simulink library "ERR_lib"  (Simulink 7.5)
settings: Solver=ode45  StartTime=0.0  StopTime=10.0  RelTol=1e-3
values from neighbouring files (symbols this model uses):
  pERR_bool_ErrDsblSwt_C = Simulink.Parameter    [ERR_par.m]
  pERR_bool_ErrIntial_C = Simulink.Parameter    [ERR_par.m]
  pERR_st_ACPTCErr_C = Simulink.Parameter    [ERR_par.m]
  pERR_st_HCUErrLampCalSt_C = Simulink.Parameter    [ERR_par.m]
  pERR_st_HCUErrLampEnbl_C = Simulink.Parameter    [ERR_par.m]
  pERR_st_HCUIntialSt_C = Simulink.Parameter    [ERR_par.m]
  pERR_st_HCUStNoErr_C = Simulink.Parameter    [ERR_par.m]
undefined symbols (not defined in the file or in its folder): p_bool_False_M, p_single_Zero_M
libraries: BaseOperationLib_Browser x64, PES_CZ_FAW x56, simulink x2
settings Model: Creator=wuaibin  LastModifiedBy=wuaibin

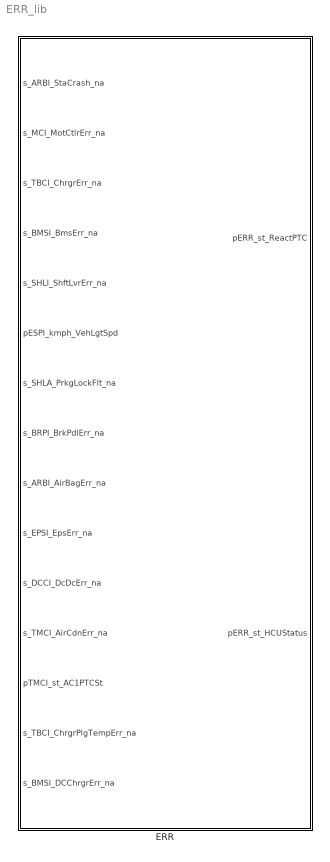
== system ERR_lib ==
  ERR : Subsystem  TreatAsAtomicUnit=on

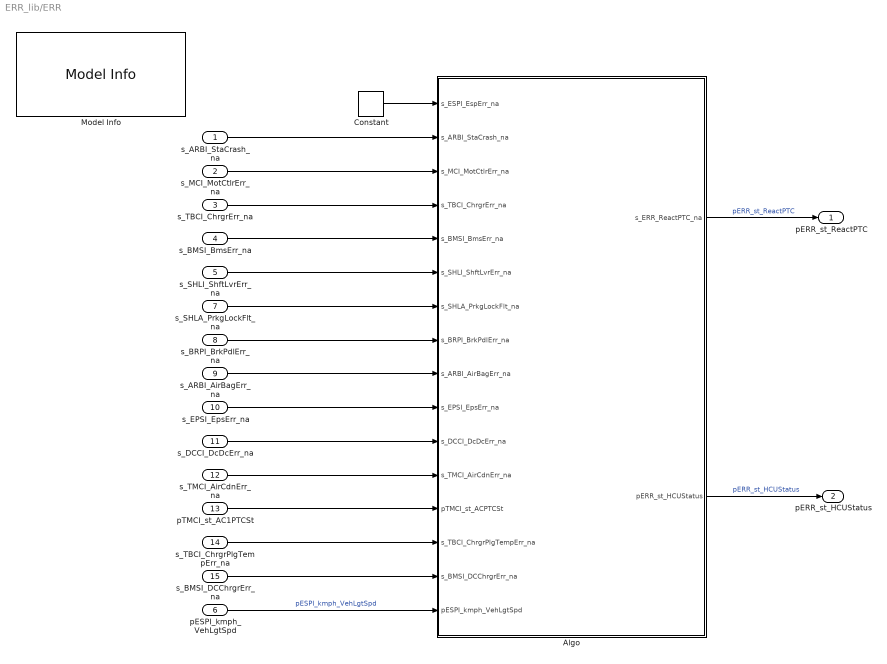
== system ERR_lib/ERR ==
  s_ARBI_StaCrash_na : Inport  PortDimensions=1
  s_MCI_MotCtlrErr_na : Inport  Port=2  PortDimensions=1
  s_TBCI_ChrgrErr_na : Inport  Port=3  PortDimensions=1
  s_BMSI_BmsErr_na : Inport  Port=4  PortDimensions=1
  s_SHLI_ShftLvrErr_na : Inport  Port=5  PortDimensions=1
  pESPI_kmph_VehLgtSpd : Inport  Port=6
  s_SHLA_PrkgLockFlt_na : Inport  Port=7  PortDimensions=1
  s_BRPI_BrkPdlErr_na : Inport  Port=8  PortDimensions=1
  s_ARBI_AirBagErr_na : Inport  Port=9  PortDimensions=1
  s_EPSI_EpsErr_na : Inport  Port=10  PortDimensions=1
  s_DCCI_DcDcErr_na : Inport  Port=11  PortDimensions=1
  s_TMCI_AirCdnErr_na : Inport  Port=12  PortDimensions=1
  pTMCI_st_AC1PTCSt : Inport  Port=13
  s_TBCI_ChrgrPlgTempErr_na : Inport  Port=14
  s_BMSI_DCChrgrErr_na : Inport  Port=15
  Algo : Subsystem
  Constant : BaseOperationLib_Browser/Sources&Sinks/Constant  Value=0  OutMin=[]  OutMax=[]  OutDataTypeMode=uint32  OutDataType=fixdt(1, 16)  ConRadixGroup=Use specified scaling  OutScaling=2^0  OutDataTypeStr=uint32
  Model Info : simulink/Model-Wide Utilities/Model Info  SystemSampleTime=-1  InitialBlockCM=None  BlockCM=None  Frame=on  DisplayStringWithTags=Model Info\nCreated: %<Created>\nCreator: wuaibin  HorizontalTextAlignment=Center  LeftAlignmentValue=0.5  SourceBlockDiagram=HQEV_HCU  TagMaxNumber=20
  pERR_st_ReactPTC : Outport  PortDimensions=1
  pERR_st_HCUStatus : Outport  Port=2
  wires:
  pESPI_kmph_VehLgtSpd/1 -> Algo/16(pESPI_kmph_VehLgtSpd)  "pESPI_kmph_VehLgtSpd"
  Constant/1 -> Algo/1(s_ESPI_EspErr_na)
  s_BMSI_DCChrgrErr_na/1 -> Algo/15(s_BMSI_DCChrgrErr_na)
  s_TBCI_ChrgrPlgTempErr_na/1 -> Algo/14(s_TBCI_ChrgrPlgTempErr_na)
  pTMCI_st_AC1PTCSt/1 -> Algo/13(pTMCI_st_ACPTCSt)
  Algo/2(pERR_st_HCUStatus) -> pERR_st_HCUStatus/1  "pERR_st_HCUStatus"
  s_ARBI_StaCrash_na/1 -> Algo/2(s_ARBI_StaCrash_na)
  s_MCI_MotCtlrErr_na/1 -> Algo/3(s_MCI_MotCtlrErr_na)
  s_TBCI_ChrgrErr_na/1 -> Algo/4(s_TBCI_ChrgrErr_na)
  s_BMSI_BmsErr_na/1 -> Algo/5(s_BMSI_BmsErr_na)
  s_SHLI_ShftLvrErr_na/1 -> Algo/6(s_SHLI_ShftLvrErr_na)
  Algo/1(s_ERR_ReactPTC_na) -> pERR_st_ReactPTC/1  "pERR_st_ReactPTC"
  s_SHLA_PrkgLockFlt_na/1 -> Algo/7(s_SHLA_PrkgLockFlt_na)
  s_BRPI_BrkPdlErr_na/1 -> Algo/8(s_BRPI_BrkPdlErr_na)
  s_ARBI_AirBagErr_na/1 -> Algo/9(s_ARBI_AirBagErr_na)
  s_EPSI_EpsErr_na/1 -> Algo/10(s_EPSI_EpsErr_na)
  s_DCCI_DcDcErr_na/1 -> Algo/11(s_DCCI_DcDcErr_na)
  s_TMCI_AirCdnErr_na/1 -> Algo/12(s_TMCI_AirCdnErr_na)

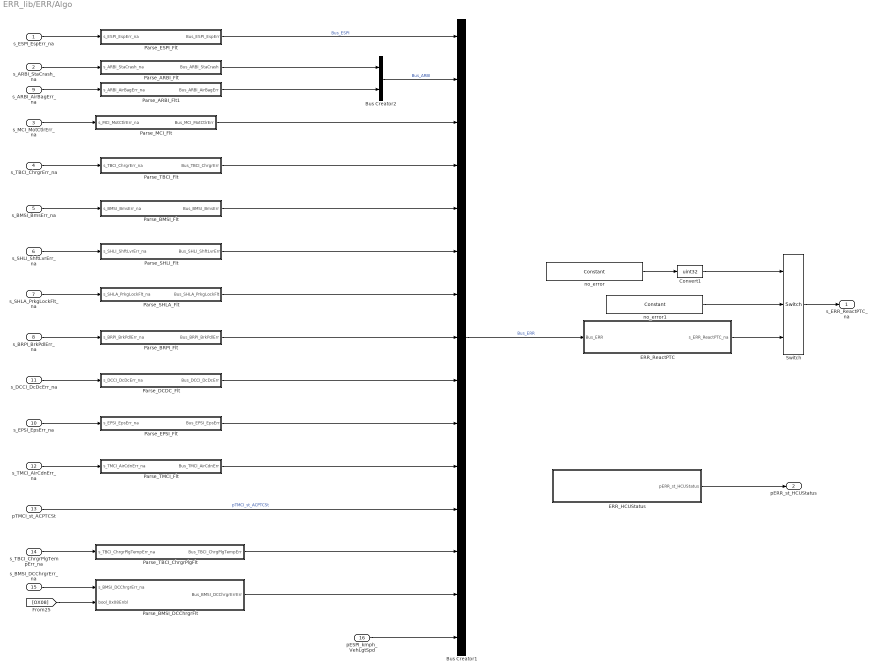
== system ERR_lib/ERR/Algo ==
  s_ESPI_EspErr_na : Inport
  s_ARBI_StaCrash_na : Inport  Port=2
  s_MCI_MotCtlrErr_na : Inport  Port=3
  s_TBCI_ChrgrErr_na : Inport  Port=4
  s_BMSI_BmsErr_na : Inport  Port=5
  s_SHLI_ShftLvrErr_na : Inport  Port=6
  s_SHLA_PrkgLockFlt_na : Inport  Port=7
  s_BRPI_BrkPdlErr_na : Inport  Port=8
  s_ARBI_AirBagErr_na : Inport  Port=9
  s_EPSI_EpsErr_na : Inport  Port=10
  s_DCCI_DcDcErr_na : Inport  Port=11
  s_TMCI_AirCdnErr_na : Inport  Port=12
  pTMCI_st_ACPTCSt : Inport  Port=13
  s_TBCI_ChrgrPlgTempErr_na : Inport  Port=14
  s_BMSI_DCChrgrErr_na : Inport  Port=15
  pESPI_kmph_VehLgtSpd : Inport  Port=16
  Bus Creator1 : BusCreator  Inputs=15
  Bus Creator2 : BusCreator  Inputs=2
  Convert1 : DataTypeConversion  OutDataTypeMode=uint32  OutDataType=fixdt(1, 16)  OutScaling=2^0  OutDataTypeStr=uint32
  ERR_HCUStatus : Subsystem
  ERR_ReactPTC : Subsystem
  Parse_ARBI_Flt : Subsystem
  Parse_ARBI_Flt1 : Subsystem
  Parse_BMSI_DCChrgrFlt : Subsystem
  Parse_BMSI_Flt : Subsystem
  Parse_BRPI_Flt : Subsystem
  Parse_DCDC_Flt : Subsystem
  Parse_EPSI_Flt : Subsystem
  Parse_ESPI_Flt : Subsystem
  Parse_MCI_Flt : Subsystem
  Parse_SHLA_Flt : Subsystem
  Parse_SHLI_Flt : Subsystem
  Parse_TBCI_ChrgrPlgFlt : Subsystem
  Parse_TBCI_Flt : Subsystem
  Parse_TMCI_Flt : Subsystem
  Switch : BaseOperationLib_Browser/Signal Routing Changed/Switch  Criteria=u2 ~= 0  Threshold=0  OutMin=[]  OutMax=[]  OutDataType=fixdt(1,16,0)  OutScaling=[]
  no_error : BaseOperationLib_Browser/Sources&Sinks/Constant  Value=pERR_bool_ErrIntial_C  OutMin=[]  OutMax=[]  OutDataType=fixdt(1, 16)  ConRadixGroup=Use specified scaling  OutScaling=2^0  OutDataTypeStr=Inherit: Inherit from 'Constant value'
  no_error1 : BaseOperationLib_Browser/Sources&Sinks/Constant  Value=pERR_bool_ErrDsblSwt_C  OutMin=[]  OutMax=[]  OutDataType=fixdt(1, 16)  ConRadixGroup=Use specified scaling  OutScaling=2^0  OutDataTypeStr=Inherit: Inherit from 'Constant value'
  s_ERR_ReactPTC_na : Outport
  pERR_st_HCUStatus : Outport  Port=2
  wires:
  pESPI_kmph_VehLgtSpd/1 -> Bus Creator1/15
  Parse_BMSI_DCChrgrFlt/1(Bus_BMSI_DCChrgrErrErr) -> Bus Creator1/14
  Parse_TBCI_ChrgrPlgFlt/1(Bus_TBCI_ChrgPlgTempErr) -> Bus Creator1/13
  [OX08] -> Parse_BMSI_DCChrgrFlt/2(bool_0x08Enbl)
  s_BMSI_DCChrgrErr_na/1 -> Parse_BMSI_DCChrgrFlt/1(s_BMSI_DCChrgrErr_na)
  s_TBCI_ChrgrPlgTempErr_na/1 -> Parse_TBCI_ChrgrPlgFlt/1(s_TBCI_ChrgrPlgTempErr_na)
  pTMCI_st_ACPTCSt/1 -> Bus Creator1/12  "pTMCI_st_ACPTCSt"
  ERR_HCUStatus/1(pERR_st_HCUStatus) -> pERR_st_HCUStatus/1
  Parse_EPSI_Flt/1(Bus_EPSI_EpsErr) -> Bus Creator1/10
  Parse_DCDC_Flt/1(Bus_DCCI_DcDcErr) -> Bus Creator1/9
  Bus Creator2/1 -> Bus Creator1/2  "Bus_ARBI"
  Parse_ARBI_Flt1/1(Bus_ARBI_AirBagErr) -> Bus Creator2/2
  Parse_BRPI_Flt/1(Bus_BRPI_BrkPdlErr) -> Bus Creator1/8
  s_BRPI_BrkPdlErr_na/1 -> Parse_BRPI_Flt/1(s_BRPI_BrkPdlErr_na)
  Parse_SHLA_Flt/1(Bus_SHLA_PrkgLockFlt) -> Bus Creator1/7
  Parse_SHLI_Flt/1(Bus_SHLI_ShftLvrErr) -> Bus Creator1/6
  Parse_BMSI_Flt/1(Bus_BMSI_BmsErr) -> Bus Creator1/5
  Parse_TBCI_Flt/1(Bus_TBCI_ChrgrErr) -> Bus Creator1/4
  Parse_MCI_Flt/1(Bus_MCI_MotCtlrErr) -> Bus Creator1/3
  Bus Creator1/1 -> ERR_ReactPTC/1(Bus_ERR)  "Bus_ERR"
  Parse_ARBI_Flt/1(Bus_ARBI_StaCrash) -> Bus Creator2/1
  Parse_ESPI_Flt/1(Bus_ESPI_EspErr) -> Bus Creator1/1  "Bus_ESPI"
  s_DCCI_DcDcErr_na/1 -> Parse_DCDC_Flt/1(s_DCCI_DcDcErr_na)
  s_EPSI_EpsErr_na/1 -> Parse_EPSI_Flt/1(s_EPSI_EpsErr_na)
  s_ARBI_AirBagErr_na/1 -> Parse_ARBI_Flt1/1(s_ARBI_AirBagErr_na)
  s_SHLA_PrkgLockFlt_na/1 -> Parse_SHLA_Flt/1(s_SHLA_PrkgLockFlt_na)
  s_SHLI_ShftLvrErr_na/1 -> Parse_SHLI_Flt/1(s_SHLI_ShftLvrErr_na)
  s_BMSI_BmsErr_na/1 -> Parse_BMSI_Flt/1(s_BMSI_BmsErr_na)
  s_TBCI_ChrgrErr_na/1 -> Parse_TBCI_Flt/1(s_TBCI_ChrgrErr_na)
  s_MCI_MotCtlrErr_na/1 -> Parse_MCI_Flt/1(s_MCI_MotCtlrErr_na)
  s_ARBI_StaCrash_na/1 -> Parse_ARBI_Flt/1(s_ARBI_StaCrash_na)
  s_ESPI_EspErr_na/1 -> Parse_ESPI_Flt/1(s_ESPI_EspErr_na)
  Switch/1 -> s_ERR_ReactPTC_na/1
  s_TMCI_AirCdnErr_na/1 -> Parse_TMCI_Flt/1(s_TMCI_AirCdnErr_na)
  Parse_TMCI_Flt/1(Bus_TMCI_AirCdnErr) -> Bus Creator1/11
  no_error/1 -> Convert1/1
  no_error1/1 -> Switch/2
  ERR_ReactPTC/1(s_ERR_ReactPTC_na) -> Switch/3
  Convert1/1 -> Switch/1

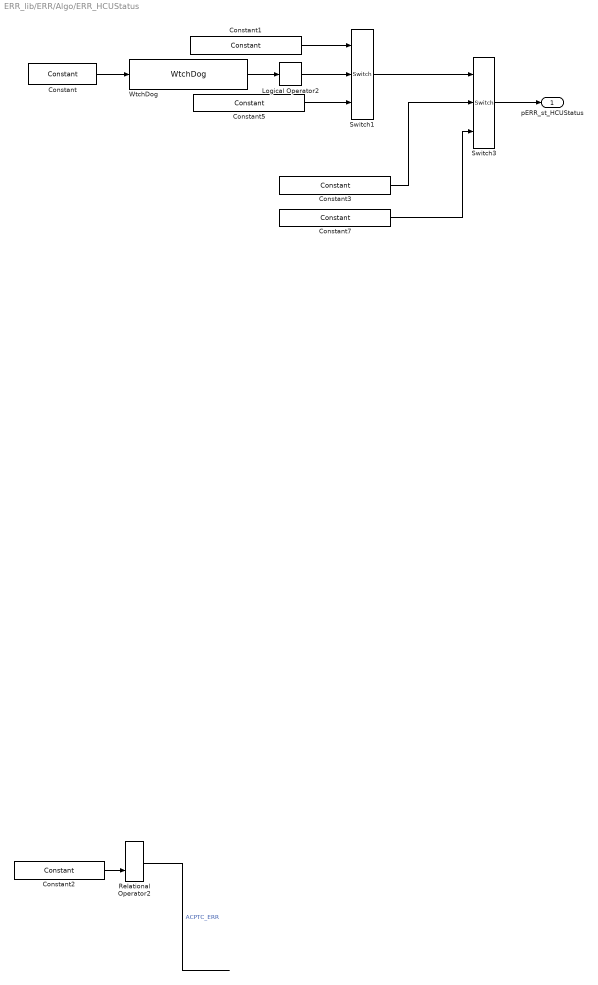
== system ERR_lib/ERR/Algo/ERR_HCUStatus ==
  Constant : BaseOperationLib_Browser/Sources&Sinks/Constant  Value=p_single_Zero_M  OutMin=[]  OutMax=[]  OutDataType=fixdt(1, 16)  ConRadixGroup=Use specified scaling  OutScaling=2^0  OutDataTypeStr=Inherit: Inherit via back propagation
  Constant1 : BaseOperationLib_Browser/Sources&Sinks/Constant  Value=pERR_st_HCUIntialSt_C  OutMin=[]  OutMax=[]  OutDataType=fixdt(1, 16)  ConRadixGroup=Use specified scaling  OutScaling=2^0  OutDataTypeStr=Inherit: Inherit from 'Constant value'
  Constant2 : BaseOperationLib_Browser/Sources&Sinks/Constant  Value=pERR_st_ACPTCErr_C  OutMin=[]  OutMax=[]  OutDataType=fixdt(1, 16)  ConRadixGroup=Use specified scaling  OutScaling=2^0  OutDataTypeStr=Inherit: Inherit from 'Constant value'
  Constant3 : BaseOperationLib_Browser/Sources&Sinks/Constant  Value=pERR_st_HCUErrLampEnbl_C  OutMin=[]  OutMax=[]  OutDataType=fixdt(1, 16)  ConRadixGroup=Use specified scaling  OutScaling=2^0  OutDataTypeStr=Inherit: Inherit from 'Constant value'
  Constant5 : BaseOperationLib_Browser/Sources&Sinks/Constant  Value=pERR_st_HCUStNoErr_C  OutMin=[]  OutMax=[]  OutDataType=fixdt(1, 16)  ConRadixGroup=Use specified scaling  OutScaling=2^0  OutDataTypeStr=Inherit: Inherit from 'Constant value'
  Constant7 : BaseOperationLib_Browser/Sources&Sinks/Constant  Value=pERR_st_HCUErrLampCalSt_C  OutMin=[]  OutMax=[]  OutDataType=fixdt(1, 16)  ConRadixGroup=Use specified scaling  OutScaling=2^0  OutDataTypeStr=Inherit: Inherit from 'Constant value'
  Logical Operator2 : BaseOperationLib_Browser/Logic Operations Changed/Logical Operator  Operator=NOT  Inputs=2  AllPortsSameDT=off  OutDataTypeMode=boolean  LogicDataType=PDT_Bool  OutDataTypeStr=boolean
  Relational Operator2 : BaseOperationLib_Browser/Logic Operations Changed/Relational Operator  Operator===  InputSameDT=on  LogicOutDataTypeMode=Specify via dialog  LogicDataType=PDT_Bool  OutDataTypeStr=PDT_Bool
  Switch1 : BaseOperationLib_Browser/Signal Routing Changed/Switch  Criteria=u2 ~= 0  Threshold=1  InputSameDT=on  OutMin=[]  OutMax=[]  OutDataType=fixdt(1,16,0)  OutScaling=[]  SaturateOnIntegerOverflow=on
  Switch3 : BaseOperationLib_Browser/Signal Routing Changed/Switch  Criteria=u2 ~= 0  Threshold=1  InputSameDT=on  OutMin=[]  OutMax=[]  OutDataType=fixdt(1,16,0)  OutScaling=[]  SaturateOnIntegerOverflow=on
  WtchDog : PES_CZ_FAW/Discontinuities/WtchDog  SystemSampleTime=-1  timeoutthres=p_ERR_WakeUpDlyTiOut_s
  pERR_st_HCUStatus : Outport
  wires:
  Relational Operator2/1 -> ?  "ACPTC_ERR"
  ? -> Relational Operator2/1
  Constant2/1 -> Relational Operator2/2
  Constant7/1 -> Switch3/3
  Constant3/1 -> Switch3/2
  Switch1/1 -> Switch3/1
  Switch3/1 -> pERR_st_HCUStatus/1
  Logical Operator2/1 -> Switch1/2
  Constant1/1 -> Switch1/1
  Constant5/1 -> Switch1/3
  WtchDog/1 -> Logical Operator2/1
  Constant/1 -> WtchDog/1

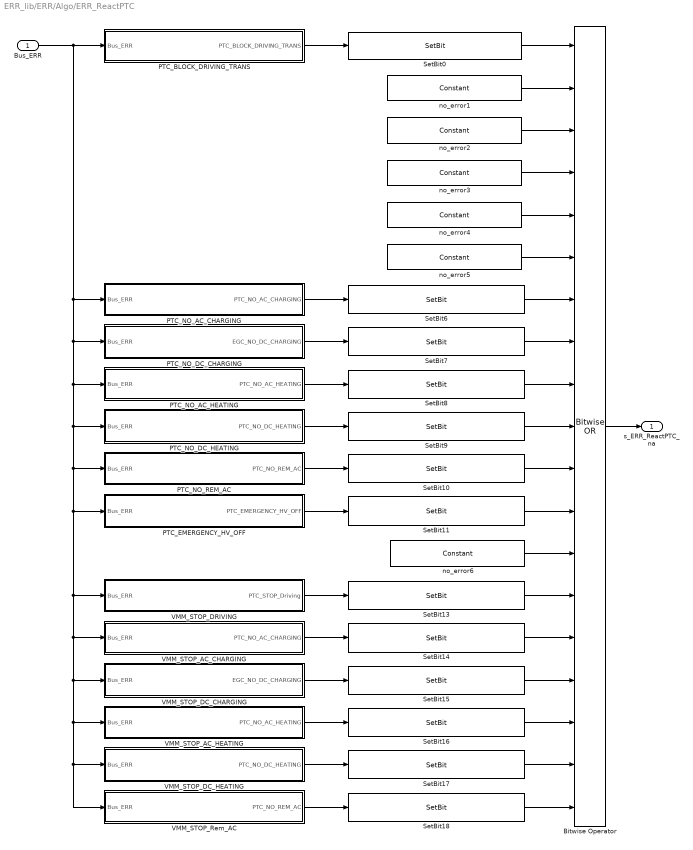
== system ERR_lib/ERR/Algo/ERR_ReactPTC ==
  Bus_ERR : Inport
  Bitwise Operator : simulink/Logic and Bit Operations/Bitwise Operator  logicop=OR  UseBitMask=off  NumInputPorts=19  BitMask=bin2dec('11011001')  BitMaskRealWorld=Stored Integer
  PTC_BLOCK_DRIVING_TRANS : Subsystem
  PTC_EMERGENCY_HV_OFF : Subsystem
  PTC_NO_AC_CHARGING : Subsystem
  PTC_NO_AC_HEATING : Subsystem
  PTC_NO_DC_CHARGING : Subsystem
  PTC_NO_DC_HEATING : Subsystem
  PTC_NO_REM_AC : Subsystem
  SetBit0 : PES_CZ_FAW/Discontinuities/SetBit  SystemSampleTime=-1  maska=FtlReactVMMTyp.BLOCK_DRIVING_TRANS
  SetBit10 : PES_CZ_FAW/Discontinuities/SetBit  SystemSampleTime=-1  maska=FtlReactVMMTyp.VMM_NO_Rem_AC
  SetBit11 : PES_CZ_FAW/Discontinuities/SetBit  SystemSampleTime=-1  maska=FtlReactVMMTyp.VMM_EMERGENCY_HV_OFF
  SetBit13 : PES_CZ_FAW/Discontinuities/SetBit  SystemSampleTime=-1  maska=FtlReactVMMTyp.VMM_STOP_DRIVING
  SetBit14 : PES_CZ_FAW/Discontinuities/SetBit  SystemSampleTime=-1  maska=FtlReactVMMTyp.VMM_STOP_AC_CHARGING
  SetBit15 : PES_CZ_FAW/Discontinuities/SetBit  SystemSampleTime=-1  maska=FtlReactVMMTyp.VMM_STOP_DC_CHARGING
  SetBit16 : PES_CZ_FAW/Discontinuities/SetBit  SystemSampleTime=-1  maska=FtlReactVMMTyp.VMM_STOP_AC_HEATING
  SetBit17 : PES_CZ_FAW/Discontinuities/SetBit  SystemSampleTime=-1  maska=FtlReactVMMTyp.VMM_STOP_DC_HEATING
  SetBit18 : PES_CZ_FAW/Discontinuities/SetBit  SystemSampleTime=-1  maska=FtlReactVMMTyp.VMM_STOP_Rem_AC
  SetBit6 : PES_CZ_FAW/Discontinuities/SetBit  SystemSampleTime=-1  maska=FtlReactVMMTyp.VMM_NO_AC_CHARGING
  SetBit7 : PES_CZ_FAW/Discontinuities/SetBit  SystemSampleTime=-1  maska=FtlReactVMMTyp.VMM_NO_DC_CHARGING
  SetBit8 : PES_CZ_FAW/Discontinuities/SetBit  SystemSampleTime=-1  maska=FtlReactVMMTyp.VMM_NO_AC_HEATING
  SetBit9 : PES_CZ_FAW/Discontinuities/SetBit  SystemSampleTime=-1  maska=FtlReactVMMTyp.VMM_NO_DC_HEATING
  VMM_STOP_AC_CHARGING : Subsystem
  VMM_STOP_AC_HEATING : Subsystem
  VMM_STOP_DC_CHARGING : Subsystem
  VMM_STOP_DC_HEATING : Subsystem
  VMM_STOP_DRIVING : Subsystem
  VMM_STOP_Rem_AC : Subsystem
  no_error{1..6} (6 alike) : BaseOperationLib_Browser/Sources&Sinks/Constant  Value=0  OutMin=[]  OutMax=[]  OutDataTypeMode=uint32  OutDataType=fixdt(1, 16)  ConRadixGroup=Use specified scaling  OutScaling=2^0  OutDataTypeStr=uint32
  s_ERR_ReactPTC_na : Outport
  wires:
  VMM_STOP_DC_CHARGING/1(EGC_NO_DC_CHARGING) -> SetBit15/1
  VMM_STOP_AC_HEATING/1(PTC_NO_AC_HEATING) -> SetBit16/1
  VMM_STOP_DC_HEATING/1(PTC_NO_DC_HEATING) -> SetBit17/1
  VMM_STOP_Rem_AC/1(PTC_NO_REM_AC) -> SetBit18/1
  VMM_STOP_AC_CHARGING/1(PTC_NO_AC_CHARGING) -> SetBit14/1
  SetBit18/1 -> Bitwise Operator/19
  SetBit17/1 -> Bitwise Operator/18
  SetBit16/1 -> Bitwise Operator/17
  SetBit15/1 -> Bitwise Operator/16
  SetBit14/1 -> Bitwise Operator/15
  SetBit13/1 -> Bitwise Operator/14
  VMM_STOP_DRIVING/1(PTC_STOP_Driving) -> SetBit13/1
  no_error6/1 -> Bitwise Operator/13
  PTC_NO_REM_AC/1(PTC_NO_REM_AC) -> SetBit10/1
  PTC_NO_DC_HEATING/1(PTC_NO_DC_HEATING) -> SetBit9/1
  PTC_NO_AC_HEATING/1(PTC_NO_AC_HEATING) -> SetBit8/1
  PTC_EMERGENCY_HV_OFF/1(PTC_EMERGENCY_HV_OFF) -> SetBit11/1
  PTC_NO_DC_CHARGING/1(EGC_NO_DC_CHARGING) -> SetBit7/1
  PTC_NO_AC_CHARGING/1(PTC_NO_AC_CHARGING) -> SetBit6/1
  SetBit11/1 -> Bitwise Operator/12
  SetBit10/1 -> Bitwise Operator/11
  SetBit9/1 -> Bitwise Operator/10
  SetBit8/1 -> Bitwise Operator/9
  SetBit7/1 -> Bitwise Operator/8
  SetBit6/1 -> Bitwise Operator/7
  Bus_ERR/1 -> PTC_BLOCK_DRIVING_TRANS/1(Bus_ERR), VMM_STOP_Rem_AC/1(Bus_ERR), VMM_STOP_DC_HEATING/1(Bus_ERR), VMM_STOP_AC_HEATING/1(Bus_ERR), VMM_STOP_DC_CHARGING/1(Bus_ERR), VMM_STOP_AC_CHARGING/1(Bus_ERR), VMM_STOP_DRIVING/1(Bus_ERR), PTC_EMERGENCY_HV_OFF/1(Bus_ERR), PTC_NO_REM_AC/1(Bus_ERR), PTC_NO_DC_HEATING/1(Bus_ERR), PTC_NO_AC_HEATING/1(Bus_ERR), PTC_NO_DC_CHARGING/1(Bus_ERR), PTC_NO_AC_CHARGING/1(Bus_ERR)
  Bitwise Operator/1 -> s_ERR_ReactPTC_na/1
  SetBit0/1 -> Bitwise Operator/1
  PTC_BLOCK_DRIVING_TRANS/1(PTC_BLOCK_DRIVING_TRANS) -> SetBit0/1
  no_error1/1 -> Bitwise Operator/2
  no_error2/1 -> Bitwise Operator/3
  no_error3/1 -> Bitwise Operator/4
  no_error4/1 -> Bitwise Operator/5
  no_error5/1 -> Bitwise Operator/6

== system ERR_lib/ERR/Algo/Parse_ARBI_Flt ==
  s_ARBI_StaCrash_na : Inport
  Bus Creator : BusCreator  Inputs=1
  GetBit : PES_CZ_FAW/Discontinuities/GetBit  SystemSampleTime=-1  maska=StaCrashTyp.CRASH
  Bus_ARBI_StaCrash : Outport
  wires:
  Bus Creator/1 -> Bus_ARBI_StaCrash/1  "Bus_ARBI_StaCrash"
  s_ARBI_StaCrash_na/1 -> GetBit/1
  GetBit/1 -> Bus Creator/1  "CRASH"

== system ERR_lib/ERR/Algo/Parse_ARBI_Flt1 ==
  s_ARBI_AirBagErr_na : Inport
  Bus Creator : BusCreator  Inputs=1
  GetBit : PES_CZ_FAW/Discontinuities/GetBit  SystemSampleTime=-1  maska=FAWAirBagErrTyp.AIRBAG_ERROR
  Bus_ARBI_AirBagErr : Outport
  wires:
  GetBit/1 -> Bus Creator/1  "AIRBAG_ERROR"
  s_ARBI_AirBagErr_na/1 -> GetBit/1
  Bus Creator/1 -> Bus_ARBI_AirBagErr/1  "Bus_ARBI_AirBagErr"

== system ERR_lib/ERR/Algo/Parse_BMSI_DCChrgrFlt ==
  s_BMSI_DCChrgrErr_na : Inport
  bool_0x08Enbl : Inport  Port=2
  Bus Creator : BusCreator  Inputs=1
  Constant17 : BaseOperationLib_Browser/Sources&Sinks/Constant  Value=p_bool_False_M  OutMin=[]  OutMax=[]  OutDataType=fixdt(1, 16)  ConRadixGroup=Use specified scaling  OutScaling=2^0  OutDataTypeStr=Inherit: Inherit via back propagation
  GetBit : PES_CZ_FAW/Discontinuities/GetBit  SystemSampleTime=-1  maska=FAWDCChrgrErr.FDC_DCChrgrErr
  Switch17 : BaseOperationLib_Browser/Signal Routing Changed/Switch  Criteria=u2 ~= 0  Threshold=1  InputSameDT=on  OutMin=[]  OutMax=[]  OutDataType=fixdt(1,16,0)  OutScaling=[]  SaturateOnIntegerOverflow=on
  Bus_BMSI_DCChrgrErrErr : Outport
  wires:
  bool_0x08Enbl/1 -> Switch17/2
  Constant17/1 -> Switch17/1
  GetBit/1 -> Switch17/3  "DCChrgrErr"
  Switch17/1 -> Bus Creator/1  "DCChrgrErrErr"
  Bus Creator/1 -> Bus_BMSI_DCChrgrErrErr/1  "Bus_BMSI_DCChrgrErrErr"
  s_BMSI_DCChrgrErr_na/1 -> GetBit/1

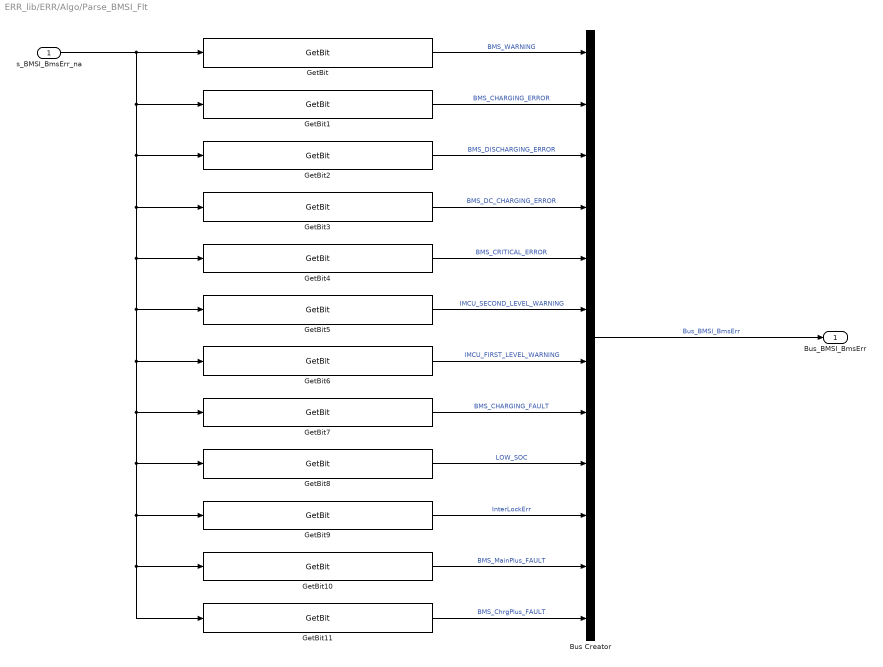
== system ERR_lib/ERR/Algo/Parse_BMSI_Flt ==
  s_BMSI_BmsErr_na : Inport
  Bus Creator : BusCreator  Inputs=12
  GetBit : PES_CZ_FAW/Discontinuities/GetBit  SystemSampleTime=-1  maska=FAWBmsErrTyp.BMS_WARNING
  GetBit1 : PES_CZ_FAW/Discontinuities/GetBit  SystemSampleTime=-1  maska=FAWBmsErrTyp.BMS_CHARGING_ERROR
  GetBit10 : PES_CZ_FAW/Discontinuities/GetBit  SystemSampleTime=-1  maska=FAWBmsErrTyp.BMS_MainPlus_FAULT
  GetBit11 : PES_CZ_FAW/Discontinuities/GetBit  SystemSampleTime=-1  maska=FAWBmsErrTyp.BMS_ChrgPlus_FAULT
  GetBit2 : PES_CZ_FAW/Discontinuities/GetBit  SystemSampleTime=-1  maska=FAWBmsErrTyp.BMS_DISCHARGING_ERROR
  GetBit3 : PES_CZ_FAW/Discontinuities/GetBit  SystemSampleTime=-1  maska=FAWBmsErrTyp.BMS_DC_CHARGING_ERROR
  GetBit4 : PES_CZ_FAW/Discontinuities/GetBit  SystemSampleTime=-1  maska=FAWBmsErrTyp.BMS_CRITICAL_ERROR
  GetBit5 : PES_CZ_FAW/Discontinuities/GetBit  SystemSampleTime=-1  maska=FAWBmsErrTyp.IMCU_SECOND_LEVEL_WARNING
  GetBit6 : PES_CZ_FAW/Discontinuities/GetBit  SystemSampleTime=-1  maska=FAWBmsErrTyp.IMCU_FIRST_LEVEL_WARNING
  GetBit7 : PES_CZ_FAW/Discontinuities/GetBit  SystemSampleTime=-1  maska=FAWBmsErrTyp.BMS_CHARGING_FAULT
  GetBit8 : PES_CZ_FAW/Discontinuities/GetBit  SystemSampleTime=-1  maska=FAWBmsErrTyp.LOW_SOC
  GetBit9 : PES_CZ_FAW/Discontinuities/GetBit  SystemSampleTime=-1  maska=FAWBmsErrTyp.InterLockErr
  Bus_BMSI_BmsErr : Outport
  wires:
  GetBit11/1 -> Bus Creator/12  "BMS_ChrgPlus_FAULT"
  GetBit10/1 -> Bus Creator/11  "BMS_MainPlus_FAULT"
  GetBit9/1 -> Bus Creator/10  "InterLockErr"
  GetBit8/1 -> Bus Creator/9  "LOW_SOC"
  GetBit7/1 -> Bus Creator/8  "BMS_CHARGING_FAULT"
  GetBit6/1 -> Bus Creator/7  "IMCU_FIRST_LEVEL_WARNING"
  GetBit5/1 -> Bus Creator/6  "IMCU_SECOND_LEVEL_WARNING"
  GetBit4/1 -> Bus Creator/5  "BMS_CRITICAL_ERROR"
  GetBit3/1 -> Bus Creator/4  "BMS_DC_CHARGING_ERROR"
  GetBit2/1 -> Bus Creator/3  "BMS_DISCHARGING_ERROR"
  GetBit1/1 -> Bus Creator/2  "BMS_CHARGING_ERROR"
  GetBit/1 -> Bus Creator/1  "BMS_WARNING"
  s_BMSI_BmsErr_na/1 -> GetBit1/1, GetBit2/1, GetBit3/1, GetBit4/1, GetBit5/1, GetBit6/1, GetBit11/1, GetBit10/1, GetBit9/1, GetBit8/1, GetBit7/1, GetBit/1
  Bus Creator/1 -> Bus_BMSI_BmsErr/1  "Bus_BMSI_BmsErr"

== system ERR_lib/ERR/Algo/Parse_BRPI_Flt ==
  s_BRPI_BrkPdlErr_na : Inport
  Bus Creator : BusCreator  Inputs=2
  GetBit : PES_CZ_FAW/Discontinuities/GetBit  SystemSampleTime=-1  maska=FAWBrkPdlErrTyp.BRAKE_STATUS_ERROR
  GetBit1 : PES_CZ_FAW/Discontinuities/GetBit  SystemSampleTime=-1  maska=FAWBrkPdlErrTyp.BRAKE_PRESSURE_SIGNAL_ERROR
  Bus_BRPI_BrkPdlErr : Outport
  wires:
  GetBit1/1 -> Bus Creator/2  "BRAKE_PRESSURE_SIGNAL_ERROR"
  Bus Creator/1 -> Bus_BRPI_BrkPdlErr/1  "Bus_BRPI_BrkPdlErr"
  s_BRPI_BrkPdlErr_na/1 -> GetBit1/1, GetBit/1
  GetBit/1 -> Bus Creator/1  "BRAKE_STATUS_ERROR"

== system ERR_lib/ERR/Algo/Parse_DCDC_Flt ==
  s_DCCI_DcDcErr_na : Inport
  Bus Creator : BusCreator  Inputs=2
  GetBit : PES_CZ_FAW/Discontinuities/GetBit  SystemSampleTime=-1  maska=FAWDcDcErrTyp.DCDC_ERROR
  GetBit1 : PES_CZ_FAW/Discontinuities/GetBit  SystemSampleTime=-1  maska=FAWDcDcErrTyp.DCDC_TEMPERATURE_INVALID
  Bus_DCCI_DcDcErr : Outport
  wires:
  GetBit1/1 -> Bus Creator/2  "DCDC_TEMPERATURE_INVALID"
  Bus Creator/1 -> Bus_DCCI_DcDcErr/1  "Bus_DCCI_DcDcErr"
  s_DCCI_DcDcErr_na/1 -> GetBit1/1, GetBit/1
  GetBit/1 -> Bus Creator/1  "DCDC_ERROR"

== system ERR_lib/ERR/Algo/Parse_EPSI_Flt ==
  s_EPSI_EpsErr_na : Inport
  Bus Creator : BusCreator  Inputs=1
  GetBit : PES_CZ_FAW/Discontinuities/GetBit  SystemSampleTime=-1  maska=FAWEpsErrTyp.EPS_ERROR
  Bus_EPSI_EpsErr : Outport
  wires:
  GetBit/1 -> Bus Creator/1  "EPS_ERROR"
  s_EPSI_EpsErr_na/1 -> GetBit/1
  Bus Creator/1 -> Bus_EPSI_EpsErr/1  "Bus_EPSI_EpsErr"

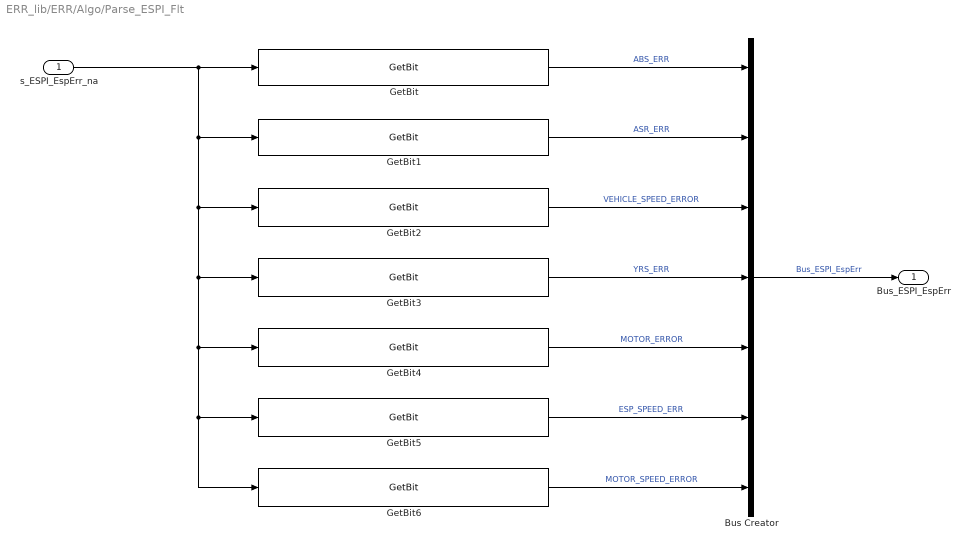
== system ERR_lib/ERR/Algo/Parse_ESPI_Flt ==
  s_ESPI_EspErr_na : Inport
  Bus Creator : BusCreator  Inputs=7
  GetBit : PES_CZ_FAW/Discontinuities/GetBit  SystemSampleTime=-1  maska=EspErrTyp.ABS_ERR
  GetBit1 : PES_CZ_FAW/Discontinuities/GetBit  SystemSampleTime=-1  maska=EspErrTyp.ASR_ERR
  GetBit2 : PES_CZ_FAW/Discontinuities/GetBit  SystemSampleTime=-1  maska=EspErrTyp.VEHICLE_SPEED_ERROR
  GetBit3 : PES_CZ_FAW/Discontinuities/GetBit  SystemSampleTime=-1  maska=EspErrTyp.YRS_ERR
  GetBit4 : PES_CZ_FAW/Discontinuities/GetBit  SystemSampleTime=-1  maska=EspErrTyp.MOTOR_ERROR
  GetBit5 : PES_CZ_FAW/Discontinuities/GetBit  SystemSampleTime=-1  maska=EspErrTyp.ESP_SPEED_ERR
  GetBit6 : PES_CZ_FAW/Discontinuities/GetBit  SystemSampleTime=-1  maska=EspErrTyp.MOTOR_SPEED_ERROR
  Bus_ESPI_EspErr : Outport
  wires:
  GetBit6/1 -> Bus Creator/7  "MOTOR_SPEED_ERROR"
  GetBit5/1 -> Bus Creator/6  "ESP_SPEED_ERR"
  GetBit/1 -> Bus Creator/1  "ABS_ERR"
  GetBit1/1 -> Bus Creator/2  "ASR_ERR"
  GetBit2/1 -> Bus Creator/3  "VEHICLE_SPEED_ERROR"
  GetBit4/1 -> Bus Creator/5  "MOTOR_ERROR"
  GetBit3/1 -> Bus Creator/4  "YRS_ERR"
  s_ESPI_EspErr_na/1 -> GetBit6/1, GetBit5/1, GetBit4/1, GetBit3/1, GetBit2/1, GetBit1/1, GetBit/1
  Bus Creator/1 -> Bus_ESPI_EspErr/1  "Bus_ESPI_EspErr"

== system ERR_lib/ERR/Algo/Parse_MCI_Flt ==
  s_MCI_MotCtlrErr_na : Inport
  Bus Creator : BusCreator  Inputs=6
  GetBit : PES_CZ_FAW/Discontinuities/GetBit  SystemSampleTime=-1  maska=MotCtrlErrTyp.MOT_WARN
  GetBit1 : PES_CZ_FAW/Discontinuities/GetBit  SystemSampleTime=-1  maska=MotCtrlErrTyp.MOT_ERR
  GetBit2 : PES_CZ_FAW/Discontinuities/GetBit  SystemSampleTime=-1  maska=MotCtrlErrTyp.MOT_WRK_STS_ERR
  GetBit3 : PES_CZ_FAW/Discontinuities/GetBit  SystemSampleTime=-1  maska=MotCtrlErrTyp.TEMPERATURE_INVALID
  GetBit4 : PES_CZ_FAW/Discontinuities/GetBit  SystemSampleTime=-1  maska=MotCtrlErrTyp.MOT_CAPACITY_V_INVALID
  GetBit5 : PES_CZ_FAW/Discontinuities/GetBit  SystemSampleTime=-1  maska=MotCtrlErrTyp.MOT_REGENERATION_ERROR
  Bus_MCI_MotCtlrErr : Outport
  wires:
  GetBit5/1 -> Bus Creator/6  "MOT_REGENERATION_ERROR"
  GetBit4/1 -> Bus Creator/5  "MOT_CAPACITY_V_INVALID"
  GetBit3/1 -> Bus Creator/4  "TEMPERATURE_INVALID"
  GetBit2/1 -> Bus Creator/3  "MOT_WRK_STS_ERR"
  GetBit1/1 -> Bus Creator/2  "MOT_ERR"
  Bus Creator/1 -> Bus_MCI_MotCtlrErr/1  "Bus_MCI_MotCtlrErr"
  s_MCI_MotCtlrErr_na/1 -> GetBit5/1, GetBit4/1, GetBit3/1, GetBit2/1, GetBit1/1, GetBit/1
  GetBit/1 -> Bus Creator/1  "MOT_WARN"

== system ERR_lib/ERR/Algo/Parse_SHLA_Flt ==
  s_SHLA_PrkgLockFlt_na : Inport
  Bus Creator : BusCreator  Inputs=1
  GetBit : PES_CZ_FAW/Discontinuities/GetBit  SystemSampleTime=-1  maska=PrkgLockFltTyp.E_PARK_PLAUSIBILITY_ERR
  Bus_SHLA_PrkgLockFlt : Outport
  wires:
  GetBit/1 -> Bus Creator/1  "E_PARK_PLAUSIBILITY_ERR"
  s_SHLA_PrkgLockFlt_na/1 -> GetBit/1
  Bus Creator/1 -> Bus_SHLA_PrkgLockFlt/1  "Bus_SHLA_PrkgLockFlt"

== system ERR_lib/ERR/Algo/Parse_SHLI_Flt ==
  s_SHLI_ShftLvrErr_na : Inport
  Bus Creator : BusCreator  Inputs=2
  GetBit : PES_CZ_FAW/Discontinuities/GetBit  SystemSampleTime=-1  maska=ShftLvrErrTyp.SHIFT_LEVER_ERROR
  GetBit1 : PES_CZ_FAW/Discontinuities/GetBit  SystemSampleTime=-1  maska=ShftLvrErrTyp.E_PARK_ERROR
  Bus_SHLI_ShftLvrErr : Outport
  wires:
  GetBit1/1 -> Bus Creator/2  "E_PARK_ERROR"
  Bus Creator/1 -> Bus_SHLI_ShftLvrErr/1  "Bus_SHLI_ShftLvrErr"
  s_SHLI_ShftLvrErr_na/1 -> GetBit1/1, GetBit/1
  GetBit/1 -> Bus Creator/1  "SHIFT_LEVER_ERROR"

== system ERR_lib/ERR/Algo/Parse_TBCI_ChrgrPlgFlt ==
  s_TBCI_ChrgrPlgTempErr_na : Inport
  Bus Creator : BusCreator  Inputs=2
  GetBit : PES_CZ_FAW/Discontinuities/GetBit  SystemSampleTime=-1  maska=ChrgrPlgTempHiErrTyp.CPT_ACPlgTempHi
  GetBit1 : PES_CZ_FAW/Discontinuities/GetBit  SystemSampleTime=-1  maska=ChrgrPlgTempHiErrTyp.CPT_DCPlgTempHi
  Bus_TBCI_ChrgPlgTempErr : Outport
  wires:
  GetBit1/1 -> Bus Creator/2  "DCPlgTempHi"
  GetBit/1 -> Bus Creator/1  "ACPlgTemHi"
  s_TBCI_ChrgrPlgTempErr_na/1 -> GetBit1/1, GetBit/1
  Bus Creator/1 -> Bus_TBCI_ChrgPlgTempErr/1  "Bus_TBCI_ChrgPlgTempErr"

== system ERR_lib/ERR/Algo/Parse_TBCI_Flt ==
  s_TBCI_ChrgrErr_na : Inport
  Bus Creator : BusCreator  Inputs=3
  GetBit : PES_CZ_FAW/Discontinuities/GetBit  SystemSampleTime=-1  maska=FAWChrgrErrTyp.CHARGER_ERROR
  GetBit1 : PES_CZ_FAW/Discontinuities/GetBit  SystemSampleTime=-1  maska=FAWChrgrErrTyp.CHARGER_ABNORMAL
  GetBit2 : PES_CZ_FAW/Discontinuities/GetBit  SystemSampleTime=-1  maska=FAWChrgrErrTyp.CHARGER_TEMPERATURE_INVALID
  Bus_TBCI_ChrgrErr : Outport
  wires:
  GetBit/1 -> Bus Creator/1  "CHARGER_ERROR"
  s_TBCI_ChrgrErr_na/1 -> GetBit/1, GetBit2/1, GetBit1/1
  Bus Creator/1 -> Bus_TBCI_ChrgrErr/1  "Bus_TBCI_ChrgrErr"
  GetBit2/1 -> Bus Creator/3  "CHARGER_TEMPERATURE_INVALID"
  GetBit1/1 -> Bus Creator/2  "CHARGER_ABNORMAL"

== system ERR_lib/ERR/Algo/Parse_TMCI_Flt ==
  s_TMCI_AirCdnErr_na : Inport
  Bus Creator : BusCreator  Inputs=1
  GetBit : PES_CZ_FAW/Discontinuities/GetBit  SystemSampleTime=-1  maska=FAWAirCdnErrTyp.AIRCDN_ERROR
  Bus_TMCI_AirCdnErr : Outport
  wires:
  Bus Creator/1 -> Bus_TMCI_AirCdnErr/1  "Bus_TMCI_AirCdnErr"
  s_TMCI_AirCdnErr_na/1 -> GetBit/1
  GetBit/1 -> Bus Creator/1  "AIRCDN_ERROR"

== system ERR_lib/ERR/Algo/ERR_ReactPTC/PTC_BLOCK_DRIVING_TRANS ==
  Bus_ERR : Inport
  Bus Selector : BusSelector  OutputSignals=Bus_BMSI_BmsErr.BMS_CRITICAL_ERROR,Bus_BMSI_BmsErr.IMCU_FIRST_LEVEL_WARNING,Bus_BMSI_BmsErr.InterLockErr
  Logical Operator : BaseOperationLib_Browser/Logic Operations Changed/Logical Operator  Operator=OR  Inputs=3  AllPortsSameDT=off  OutDataTypeMode=boolean  LogicDataType=PDT_Bool  OutDataTypeStr=boolean
  PTC_BLOCK_DRIVING_TRANS : Outport
  wires:
  Bus Selector/3 -> Logical Operator/3  "<InterLockErr>"
  Bus Selector/2 -> Logical Operator/2  "<IMCU_FIRST_LEVEL_WARNING>"
  Bus Selector/1 -> Logical Operator/1  "<BMS_CRITICAL_ERROR>"
  Logical Operator/1 -> PTC_BLOCK_DRIVING_TRANS/1
  Bus_ERR/1 -> Bus Selector/1

== system ERR_lib/ERR/Algo/ERR_ReactPTC/PTC_EMERGENCY_HV_OFF ==
  Bus_ERR : Inport
  Bus Selector : BusSelector  OutputSignals=Bus_BMSI_BmsErr.BMS_CRITICAL_ERROR,Bus_ARBI.Bus_ARBI_StaCrash.CRASH
  Logical Operator : BaseOperationLib_Browser/Logic Operations Changed/Logical Operator  Operator=OR  Inputs=2  AllPortsSameDT=off  OutDataTypeMode=boolean  LogicDataType=PDT_Bool  OutDataTypeStr=boolean
  PTC_EMERGENCY_HV_OFF : Outport
  wires:
  Bus Selector/2 -> Logical Operator/2  "<CRASH>"
  Bus Selector/1 -> Logical Operator/1  "<BMS_CRITICAL_ERROR>"
  Logical Operator/1 -> PTC_EMERGENCY_HV_OFF/1
  Bus_ERR/1 -> Bus Selector/1

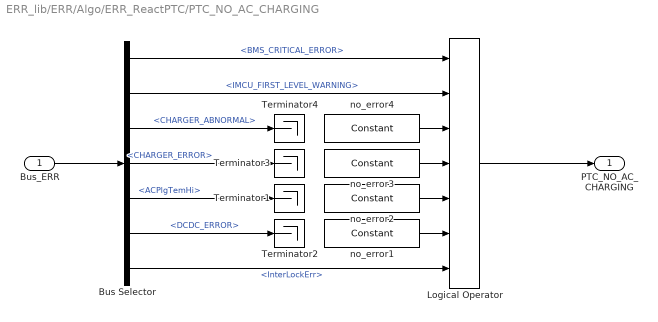
== system ERR_lib/ERR/Algo/ERR_ReactPTC/PTC_NO_AC_CHARGING ==
  Bus_ERR : Inport
  Bus Selector : BusSelector  OutputSignals=Bus_BMSI_BmsErr.BMS_CRITICAL_ERROR,Bus_BMSI_BmsErr.IMCU_FIRST_LEVEL_WARNING,Bus_TBCI_ChrgrErr.CHARGER_ABNORMAL,Bus_TBCI_ChrgrErr.CHARGER_ERROR,Bus_TBCI_ChrgPlgTempErr.ACPlgTemHi,Bus_DCCI_DcDcErr.DCDC_ERROR,Bus_BMSI_BmsErr.InterLockErr
  Logical Operator : BaseOperationLib_Browser/Logic Operations Changed/Logical Operator  Operator=OR  Inputs=7  AllPortsSameDT=off  OutDataTypeMode=boolean  LogicDataType=PDT_Bool  OutDataTypeStr=boolean
  Terminator{1..4} (4 alike) : Terminator
  no_error{1..4} (4 alike) : BaseOperationLib_Browser/Sources&Sinks/Constant  Value=p_bool_False_M  OutMin=[]  OutMax=[]  OutDataType=fixdt(1, 16)  ConRadixGroup=Use specified scaling  OutScaling=2^0  OutDataTypeStr=Inherit: Inherit from 'Constant value'
  PTC_NO_AC_CHARGING : Outport
  wires:
  Bus Selector/7 -> Logical Operator/7  "<InterLockErr>"
  Bus Selector/2 -> Logical Operator/2  "<IMCU_FIRST_LEVEL_WARNING>"
  Bus_ERR/1 -> Bus Selector/1
  Logical Operator/1 -> PTC_NO_AC_CHARGING/1
  Bus Selector/1 -> Logical Operator/1  "<BMS_CRITICAL_ERROR>"
  Bus Selector/5 -> Terminator1/1  "<ACPlgTemHi>"
  no_error2/1 -> Logical Operator/5
  no_error1/1 -> Logical Operator/6
  Bus Selector/6 -> Terminator2/1  "<DCDC_ERROR>"
  Bus Selector/4 -> Terminator3/1  "<CHARGER_ERROR>"
  no_error3/1 -> Logical Operator/4
  no_error4/1 -> Logical Operator/3
  Bus Selector/3 -> Terminator4/1  "<CHARGER_ABNORMAL>"

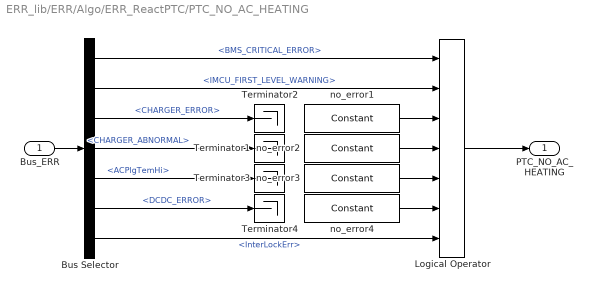
== system ERR_lib/ERR/Algo/ERR_ReactPTC/PTC_NO_AC_HEATING ==
  Bus_ERR : Inport
  Bus Selector : BusSelector  OutputSignals=Bus_BMSI_BmsErr.BMS_CRITICAL_ERROR,Bus_BMSI_BmsErr.IMCU_FIRST_LEVEL_WARNING,Bus_TBCI_ChrgrErr.CHARGER_ERROR,Bus_TBCI_ChrgrErr.CHARGER_ABNORMAL,Bus_TBCI_ChrgPlgTempErr.ACPlgTemHi,Bus_DCCI_DcDcErr.DCDC_ERROR,Bus_BMSI_BmsErr.InterLockErr
  Logical Operator : BaseOperationLib_Browser/Logic Operations Changed/Logical Operator  Operator=OR  Inputs=7  AllPortsSameDT=off  OutDataTypeMode=boolean  LogicDataType=PDT_Bool  OutDataTypeStr=boolean
  Terminator{1..4} (4 alike) : Terminator
  no_error{1..4} (4 alike) : BaseOperationLib_Browser/Sources&Sinks/Constant  Value=p_bool_False_M  OutMin=[]  OutMax=[]  OutDataType=fixdt(1, 16)  ConRadixGroup=Use specified scaling  OutScaling=2^0  OutDataTypeStr=Inherit: Inherit from 'Constant value'
  PTC_NO_AC_HEATING : Outport
  wires:
  Bus Selector/7 -> Logical Operator/7  "<InterLockErr>"
  Bus Selector/2 -> Logical Operator/2  "<IMCU_FIRST_LEVEL_WARNING>"
  Bus Selector/1 -> Logical Operator/1  "<BMS_CRITICAL_ERROR>"
  Logical Operator/1 -> PTC_NO_AC_HEATING/1
  Bus_ERR/1 -> Bus Selector/1
  no_error1/1 -> Logical Operator/3
  Bus Selector/3 -> Terminator2/1  "<CHARGER_ERROR>"
  no_error2/1 -> Logical Operator/4
  Bus Selector/4 -> Terminator1/1  "<CHARGER_ABNORMAL>"
  no_error3/1 -> Logical Operator/5
  Bus Selector/5 -> Terminator3/1  "<ACPlgTemHi>"
  Bus Selector/6 -> Terminator4/1  "<DCDC_ERROR>"
  no_error4/1 -> Logical Operator/6

== system ERR_lib/ERR/Algo/ERR_ReactPTC/PTC_NO_DC_CHARGING ==
  Bus_ERR : Inport
  Bus Selector : BusSelector  OutputSignals=Bus_BMSI_BmsErr.BMS_DC_CHARGING_ERROR,Bus_BMSI_BmsErr.BMS_CRITICAL_ERROR,Bus_BMSI_BmsErr.IMCU_FIRST_LEVEL_WARNING,Bus_TBCI_ChrgPlgTempErr.DCPlgTempHi,Bus_BMSI_DCChrgrErrErr.DCChrgrErrErr,Bus_BMSI_BmsErr.InterLockErr
  Logical Operator : BaseOperationLib_Browser/Logic Operations Changed/Logical Operator  Operator=OR  Inputs=6  AllPortsSameDT=off  OutDataTypeMode=boolean  LogicDataType=PDT_Bool  OutDataTypeStr=boolean
  Terminator1 : Terminator
  Terminator4 : Terminator
  no_error2 : BaseOperationLib_Browser/Sources&Sinks/Constant  Value=p_bool_False_M  OutMin=[]  OutMax=[]  OutDataType=fixdt(1, 16)  ConRadixGroup=Use specified scaling  OutScaling=2^0  OutDataTypeStr=Inherit: Inherit from 'Constant value'
  no_error4 : BaseOperationLib_Browser/Sources&Sinks/Constant  Value=p_bool_False_M  OutMin=[]  OutMax=[]  OutDataType=fixdt(1, 16)  ConRadixGroup=Use specified scaling  OutScaling=2^0  OutDataTypeStr=Inherit: Inherit from 'Constant value'
  EGC_NO_DC_CHARGING : Outport
  wires:
  Bus Selector/6 -> Logical Operator/6  "<InterLockErr>"
  Bus Selector/5 -> Logical Operator/5  "<DCChrgrErrErr>"
  Bus Selector/2 -> Logical Operator/2  "<BMS_CRITICAL_ERROR>"
  Bus_ERR/1 -> Bus Selector/1
  Logical Operator/1 -> EGC_NO_DC_CHARGING/1
  Bus Selector/1 -> Terminator4/1  "<BMS_DC_CHARGING_ERROR>"
  no_error4/1 -> Logical Operator/1
  Bus Selector/3 -> Logical Operator/3  "<IMCU_FIRST_LEVEL_WARNING>"
  no_error2/1 -> Logical Operator/4
  Bus Selector/4 -> Terminator1/1  "<DCPlgTempHi>"

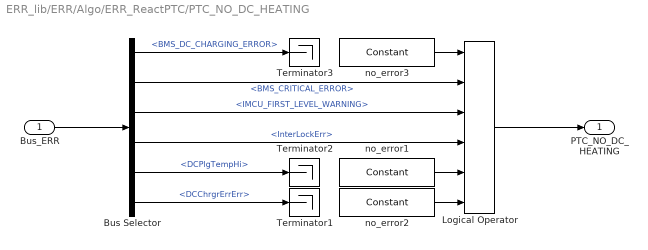
== system ERR_lib/ERR/Algo/ERR_ReactPTC/PTC_NO_DC_HEATING ==
  Bus_ERR : Inport
  Bus Selector : BusSelector  OutputSignals=Bus_BMSI_BmsErr.BMS_DC_CHARGING_ERROR,Bus_BMSI_BmsErr.BMS_CRITICAL_ERROR,Bus_BMSI_BmsErr.IMCU_FIRST_LEVEL_WARNING,Bus_BMSI_BmsErr.InterLockErr,Bus_TBCI_ChrgPlgTempErr.DCPlgTempHi,Bus_BMSI_DCChrgrErrErr.DCChrgrErrErr
  Logical Operator : BaseOperationLib_Browser/Logic Operations Changed/Logical Operator  Operator=OR  Inputs=6  AllPortsSameDT=off  OutDataTypeMode=boolean  LogicDataType=PDT_Bool  OutDataTypeStr=boolean
  Terminator1 : Terminator
  Terminator2 : Terminator
  Terminator3 : Terminator
  no_error1 : BaseOperationLib_Browser/Sources&Sinks/Constant  Value=p_bool_False_M  OutMin=[]  OutMax=[]  OutDataType=fixdt(1, 16)  ConRadixGroup=Use specified scaling  OutScaling=2^0  OutDataTypeStr=Inherit: Inherit from 'Constant value'
  no_error2 : BaseOperationLib_Browser/Sources&Sinks/Constant  Value=p_bool_False_M  OutMin=[]  OutMax=[]  OutDataType=fixdt(1, 16)  ConRadixGroup=Use specified scaling  OutScaling=2^0  OutDataTypeStr=Inherit: Inherit from 'Constant value'
  no_error3 : BaseOperationLib_Browser/Sources&Sinks/Constant  Value=p_bool_False_M  OutMin=[]  OutMax=[]  OutDataType=fixdt(1, 16)  ConRadixGroup=Use specified scaling  OutScaling=2^0  OutDataTypeStr=Inherit: Inherit from 'Constant value'
  PTC_NO_DC_HEATING : Outport
  wires:
  Bus Selector/4 -> Logical Operator/4  "<InterLockErr>"
  Bus Selector/3 -> Logical Operator/3  "<IMCU_FIRST_LEVEL_WARNING>"
  Bus Selector/2 -> Logical Operator/2  "<BMS_CRITICAL_ERROR>"
  Logical Operator/1 -> PTC_NO_DC_HEATING/1
  Bus_ERR/1 -> Bus Selector/1
  no_error1/1 -> Logical Operator/5
  Bus Selector/5 -> Terminator2/1  "<DCPlgTempHi>"
  Bus Selector/6 -> Terminator1/1  "<DCChrgrErrErr>"
  no_error2/1 -> Logical Operator/6
  no_error3/1 -> Logical Operator/1
  Bus Selector/1 -> Terminator3/1  "<BMS_DC_CHARGING_ERROR>"

== system ERR_lib/ERR/Algo/ERR_ReactPTC/PTC_NO_REM_AC ==
  Bus_ERR : Inport
  Bus Selector : BusSelector  OutputSignals=Bus_BMSI_BmsErr.BMS_CRITICAL_ERROR,Bus_BMSI_BmsErr.IMCU_FIRST_LEVEL_WARNING,Bus_TMCI_AirCdnErr.AIRCDN_ERROR
  Logical Operator : BaseOperationLib_Browser/Logic Operations Changed/Logical Operator  Operator=OR  Inputs=3  AllPortsSameDT=off  OutDataTypeMode=boolean  LogicDataType=PDT_Bool  OutDataTypeStr=boolean
  PTC_NO_REM_AC : Outport
  wires:
  Bus Selector/3 -> Logical Operator/3  "<AIRCDN_ERROR>"
  Bus Selector/2 -> Logical Operator/2  "<IMCU_FIRST_LEVEL_WARNING>"
  Bus Selector/1 -> Logical Operator/1  "<BMS_CRITICAL_ERROR>"
  Logical Operator/1 -> PTC_NO_REM_AC/1
  Bus_ERR/1 -> Bus Selector/1

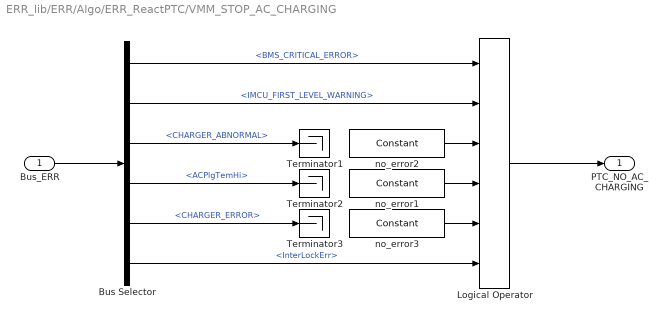
== system ERR_lib/ERR/Algo/ERR_ReactPTC/VMM_STOP_AC_CHARGING ==
  Bus_ERR : Inport
  Bus Selector : BusSelector  OutputSignals=Bus_BMSI_BmsErr.BMS_CRITICAL_ERROR,Bus_BMSI_BmsErr.IMCU_FIRST_LEVEL_WARNING,Bus_TBCI_ChrgrErr.CHARGER_ABNORMAL,Bus_TBCI_ChrgPlgTempErr.ACPlgTemHi,Bus_TBCI_ChrgrErr.CHARGER_ERROR,Bus_BMSI_BmsErr.InterLockErr
  Logical Operator : BaseOperationLib_Browser/Logic Operations Changed/Logical Operator  Operator=OR  Inputs=6  AllPortsSameDT=off  OutDataTypeMode=boolean  LogicDataType=PDT_Bool  OutDataTypeStr=boolean
  Terminator1 : Terminator
  Terminator2 : Terminator
  Terminator3 : Terminator
  no_error1 : BaseOperationLib_Browser/Sources&Sinks/Constant  Value=p_bool_False_M  OutMin=[]  OutMax=[]  OutDataType=fixdt(1, 16)  ConRadixGroup=Use specified scaling  OutScaling=2^0  OutDataTypeStr=Inherit: Inherit from 'Constant value'
  no_error2 : BaseOperationLib_Browser/Sources&Sinks/Constant  Value=p_bool_False_M  OutMin=[]  OutMax=[]  OutDataType=fixdt(1, 16)  ConRadixGroup=Use specified scaling  OutScaling=2^0  OutDataTypeStr=Inherit: Inherit from 'Constant value'
  no_error3 : BaseOperationLib_Browser/Sources&Sinks/Constant  Value=p_bool_False_M  OutMin=[]  OutMax=[]  OutDataType=fixdt(1, 16)  ConRadixGroup=Use specified scaling  OutScaling=2^0  OutDataTypeStr=Inherit: Inherit from 'Constant value'
  PTC_NO_AC_CHARGING : Outport
  wires:
  Bus Selector/6 -> Logical Operator/6  "<InterLockErr>"
  Bus Selector/2 -> Logical Operator/2  "<IMCU_FIRST_LEVEL_WARNING>"
  Bus Selector/1 -> Logical Operator/1  "<BMS_CRITICAL_ERROR>"
  Logical Operator/1 -> PTC_NO_AC_CHARGING/1
  Bus_ERR/1 -> Bus Selector/1
  no_error2/1 -> Logical Operator/3
  Bus Selector/3 -> Terminator1/1  "<CHARGER_ABNORMAL>"
  Bus Selector/4 -> Terminator2/1  "<ACPlgTemHi>"
  no_error1/1 -> Logical Operator/4
  Bus Selector/5 -> Terminator3/1  "<CHARGER_ERROR>"
  no_error3/1 -> Logical Operator/5

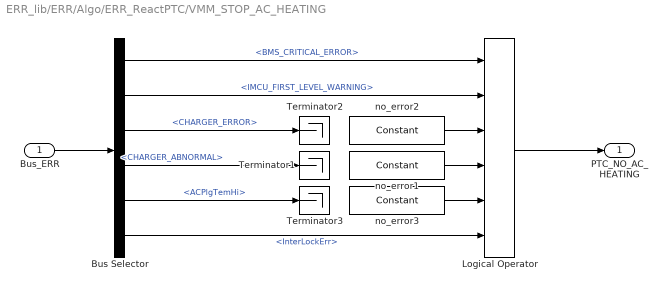
== system ERR_lib/ERR/Algo/ERR_ReactPTC/VMM_STOP_AC_HEATING ==
  Bus_ERR : Inport
  Bus Selector : BusSelector  OutputSignals=Bus_BMSI_BmsErr.BMS_CRITICAL_ERROR,Bus_BMSI_BmsErr.IMCU_FIRST_LEVEL_WARNING,Bus_TBCI_ChrgrErr.CHARGER_ERROR,Bus_TBCI_ChrgrErr.CHARGER_ABNORMAL,Bus_TBCI_ChrgPlgTempErr.ACPlgTemHi,Bus_BMSI_BmsErr.InterLockErr
  Logical Operator : BaseOperationLib_Browser/Logic Operations Changed/Logical Operator  Operator=OR  Inputs=6  AllPortsSameDT=off  OutDataTypeMode=boolean  LogicDataType=PDT_Bool  OutDataTypeStr=boolean
  Terminator1 : Terminator
  Terminator2 : Terminator
  Terminator3 : Terminator
  no_error1 : BaseOperationLib_Browser/Sources&Sinks/Constant  Value=p_bool_False_M  OutMin=[]  OutMax=[]  OutDataType=fixdt(1, 16)  ConRadixGroup=Use specified scaling  OutScaling=2^0  OutDataTypeStr=Inherit: Inherit from 'Constant value'
  no_error2 : BaseOperationLib_Browser/Sources&Sinks/Constant  Value=p_bool_False_M  OutMin=[]  OutMax=[]  OutDataType=fixdt(1, 16)  ConRadixGroup=Use specified scaling  OutScaling=2^0  OutDataTypeStr=Inherit: Inherit from 'Constant value'
  no_error3 : BaseOperationLib_Browser/Sources&Sinks/Constant  Value=p_bool_False_M  OutMin=[]  OutMax=[]  OutDataType=fixdt(1, 16)  ConRadixGroup=Use specified scaling  OutScaling=2^0  OutDataTypeStr=Inherit: Inherit from 'Constant value'
  PTC_NO_AC_HEATING : Outport
  wires:
  Bus Selector/6 -> Logical Operator/6  "<InterLockErr>"
  Bus Selector/2 -> Logical Operator/2  "<IMCU_FIRST_LEVEL_WARNING>"
  Bus Selector/1 -> Logical Operator/1  "<BMS_CRITICAL_ERROR>"
  Bus_ERR/1 -> Bus Selector/1
  Logical Operator/1 -> PTC_NO_AC_HEATING/1
  no_error3/1 -> Logical Operator/5
  Bus Selector/5 -> Terminator3/1  "<ACPlgTemHi>"
  no_error1/1 -> Logical Operator/4
  Bus Selector/4 -> Terminator1/1  "<CHARGER_ABNORMAL>"
  no_error2/1 -> Logical Operator/3
  Bus Selector/3 -> Terminator2/1  "<CHARGER_ERROR>"

== system ERR_lib/ERR/Algo/ERR_ReactPTC/VMM_STOP_DC_CHARGING ==
  Bus_ERR : Inport
  Bus Selector : BusSelector  OutputSignals=Bus_BMSI_BmsErr.BMS_DC_CHARGING_ERROR,Bus_BMSI_BmsErr.BMS_CRITICAL_ERROR,Bus_BMSI_BmsErr.IMCU_FIRST_LEVEL_WARNING,Bus_TBCI_ChrgPlgTempErr.DCPlgTempHi,Bus_BMSI_DCChrgrErrErr.DCChrgrErrErr,Bus_BMSI_BmsErr.InterLockErr
  Logical Operator : BaseOperationLib_Browser/Logic Operations Changed/Logical Operator  Operator=OR  Inputs=6  AllPortsSameDT=off  OutDataTypeMode=boolean  LogicDataType=PDT_Bool  OutDataTypeStr=boolean
  Terminator1 : Terminator
  Terminator2 : Terminator
  Terminator3 : Terminator
  no_error1 : BaseOperationLib_Browser/Sources&Sinks/Constant  Value=p_bool_False_M  OutMin=[]  OutMax=[]  OutDataType=fixdt(1, 16)  ConRadixGroup=Use specified scaling  OutScaling=2^0  OutDataTypeStr=Inherit: Inherit from 'Constant value'
  no_error2 : BaseOperationLib_Browser/Sources&Sinks/Constant  Value=p_bool_False_M  OutMin=[]  OutMax=[]  OutDataType=fixdt(1, 16)  ConRadixGroup=Use specified scaling  OutScaling=2^0  OutDataTypeStr=Inherit: Inherit from 'Constant value'
  no_error3 : BaseOperationLib_Browser/Sources&Sinks/Constant  Value=p_bool_False_M  OutMin=[]  OutMax=[]  OutDataType=fixdt(1, 16)  ConRadixGroup=Use specified scaling  OutScaling=2^0  OutDataTypeStr=Inherit: Inherit from 'Constant value'
  EGC_NO_DC_CHARGING : Outport
  wires:
  Bus Selector/6 -> Logical Operator/6  "<InterLockErr>"
  Bus Selector/3 -> Logical Operator/3  "<IMCU_FIRST_LEVEL_WARNING>"
  Bus Selector/2 -> Logical Operator/2  "<BMS_CRITICAL_ERROR>"
  Logical Operator/1 -> EGC_NO_DC_CHARGING/1
  Bus_ERR/1 -> Bus Selector/1
  no_error3/1 -> Logical Operator/1
  Bus Selector/1 -> Terminator3/1  "<BMS_DC_CHARGING_ERROR>"
  no_error1/1 -> Logical Operator/4
  Bus Selector/4 -> Terminator1/1  "<DCPlgTempHi>"
  no_error2/1 -> Logical Operator/5
  Bus Selector/5 -> Terminator2/1  "<DCChrgrErrErr>"

== system ERR_lib/ERR/Algo/ERR_ReactPTC/VMM_STOP_DC_HEATING ==
  Bus_ERR : Inport
  Bus Selector : BusSelector  OutputSignals=Bus_BMSI_BmsErr.BMS_DC_CHARGING_ERROR,Bus_BMSI_BmsErr.BMS_CRITICAL_ERROR,Bus_BMSI_BmsErr.IMCU_FIRST_LEVEL_WARNING,Bus_BMSI_BmsErr.InterLockErr,Bus_TBCI_ChrgPlgTempErr.DCPlgTempHi,Bus_BMSI_DCChrgrErrErr.DCChrgrErrErr
  Logical Operator : BaseOperationLib_Browser/Logic Operations Changed/Logical Operator  Operator=OR  Inputs=6  AllPortsSameDT=off  OutDataTypeMode=boolean  LogicDataType=PDT_Bool  OutDataTypeStr=boolean
  Terminator : Terminator
  Terminator1 : Terminator
  Terminator3 : Terminator
  no_error1 : BaseOperationLib_Browser/Sources&Sinks/Constant  Value=p_bool_False_M  OutMin=[]  OutMax=[]  OutDataType=fixdt(1, 16)  ConRadixGroup=Use specified scaling  OutScaling=2^0  OutDataTypeStr=Inherit: Inherit from 'Constant value'
  no_error2 : BaseOperationLib_Browser/Sources&Sinks/Constant  Value=p_bool_False_M  OutMin=[]  OutMax=[]  OutDataType=fixdt(1, 16)  ConRadixGroup=Use specified scaling  OutScaling=2^0  OutDataTypeStr=Inherit: Inherit from 'Constant value'
  no_error3 : BaseOperationLib_Browser/Sources&Sinks/Constant  Value=p_bool_False_M  OutMin=[]  OutMax=[]  OutDataType=fixdt(1, 16)  ConRadixGroup=Use specified scaling  OutScaling=2^0  OutDataTypeStr=Inherit: Inherit from 'Constant value'
  PTC_NO_DC_HEATING : Outport
  wires:
  Bus Selector/4 -> Logical Operator/4  "<InterLockErr>"
  Bus Selector/3 -> Logical Operator/3  "<IMCU_FIRST_LEVEL_WARNING>"
  Bus Selector/2 -> Logical Operator/2  "<BMS_CRITICAL_ERROR>"
  Bus_ERR/1 -> Bus Selector/1
  Logical Operator/1 -> PTC_NO_DC_HEATING/1
  no_error3/1 -> Logical Operator/6
  Bus Selector/6 -> Terminator3/1  "<DCChrgrErrErr>"
  Bus Selector/5 -> Terminator1/1  "<DCPlgTempHi>"
  no_error1/1 -> Logical Operator/5
  Bus Selector/1 -> Terminator/1  "<BMS_DC_CHARGING_ERROR>"
  no_error2/1 -> Logical Operator/1

== system ERR_lib/ERR/Algo/ERR_ReactPTC/VMM_STOP_DRIVING ==
  Bus_ERR : Inport
  Bus Selector : BusSelector  OutputSignals=Bus_MCI_MotCtlrErr.MOT_ERR,Bus_BMSI_BmsErr.InterLockErr,pESPI_kmph_VehLgtSpd
  Constant : BaseOperationLib_Browser/Sources&Sinks/Constant  Value=3  OutMin=[]  OutMax=[]  OutDataTypeMode=single  OutDataType=fixdt(1, 16)  ConRadixGroup=Use specified scaling  OutScaling=2^0  OutDataTypeStr=single
  Logical Operator : BaseOperationLib_Browser/Logic Operations Changed/Logical Operator  Operator=OR  Inputs=2  AllPortsSameDT=off  OutDataTypeMode=boolean  LogicDataType=PDT_Bool  OutDataTypeStr=boolean
  Logical Operator1 : BaseOperationLib_Browser/Logic Operations Changed/Logical Operator  Operator=AND  Inputs=2  AllPortsSameDT=on  OutDataTypeMode=Specify via dialog  LogicDataType=PDT_Bool  OutDataTypeStr=PDT_Bool
  Relational Operator : BaseOperationLib_Browser/Logic Operations Changed/Relational Operator  Operator=<=  InputSameDT=on  LogicOutDataTypeMode=Specify via dialog  LogicDataType=PDT_Bool  OutDataTypeStr=PDT_Bool
  Terminator1 : Terminator
  no_error2 : BaseOperationLib_Browser/Sources&Sinks/Constant  Value=p_bool_False_M  OutMin=[]  OutMax=[]  OutDataType=fixdt(1, 16)  ConRadixGroup=Use specified scaling  OutScaling=2^0  OutDataTypeStr=Inherit: Inherit from 'Constant value'
  PTC_STOP_Driving : Outport
  wires:
  Logical Operator1/1 -> Logical Operator/2
  Relational Operator/1 -> Logical Operator1/2
  Bus Selector/2 -> Logical Operator1/1  "<InterLockErr>"
  Constant/1 -> Relational Operator/2
  Bus Selector/3 -> Relational Operator/1  "<pESPI_kmph_VehLgtSpd>"
  Logical Operator/1 -> PTC_STOP_Driving/1
  Bus_ERR/1 -> Bus Selector/1
  no_error2/1 -> Logical Operator/1
  Bus Selector/1 -> Terminator1/1  "<MOT_ERR>"

== system ERR_lib/ERR/Algo/ERR_ReactPTC/VMM_STOP_Rem_AC ==
  Bus_ERR : Inport
  Bus Selector : BusSelector  OutputSignals=Bus_BMSI_BmsErr.BMS_CRITICAL_ERROR,Bus_BMSI_BmsErr.IMCU_FIRST_LEVEL_WARNING,Bus_TMCI_AirCdnErr.AIRCDN_ERROR
  Logical Operator : BaseOperationLib_Browser/Logic Operations Changed/Logical Operator  Operator=OR  Inputs=3  AllPortsSameDT=off  OutDataTypeMode=boolean  LogicDataType=PDT_Bool  OutDataTypeStr=boolean
  PTC_NO_REM_AC : Outport
  wires:
  Bus Selector/3 -> Logical Operator/3  "<AIRCDN_ERROR>"
  Bus Selector/2 -> Logical Operator/2  "<IMCU_FIRST_LEVEL_WARNING>"
  Bus Selector/1 -> Logical Operator/1  "<BMS_CRITICAL_ERROR>"
  Bus_ERR/1 -> Bus Selector/1
  Logical Operator/1 -> PTC_NO_REM_AC/1
